simulink model "EZQ4sLStEnCtrl"  (R2018b)
settings: Solver=FixedStepDiscrete  StartTime=0.0  StopTime=20  FixedStep=0.01  RelTol=1e-3
undefined symbols (not defined in the file or in its folder): data, KeSMSw4SAcsMdSecRwLtStBkReclnRstTm_Val, KeSMSw4SSecRwLtStLgrstOtwdInwdClosePos1_Val, KeSMSw4SSecRwLtStLgrstUpwdDnwdClosePos1_Val, KeSMSw4SSecRwLtStLgrstUpwdDnwdClosePos2_Val, SecRwLtStBkReclnEn_Clear, SecRwLtStBkReclnEn_Set, SecRwLtStFtrstEn_Clear, SecRwLtStFtrstEn_Set, SecRwLtStFwdBkwdEn_Clear, SecRwLtStFwdBkwdEn_Set, SecRwLtStLgrstInwdOtwdEn_Clear, SecRwLtStLgrstInwdOtwdEn_Set, SecRwLtStLgrstUpwdDnwdEn_Clear, SecRwLtStLgrstUpwdDnwdEn_Set
libraries: simulink x1
settings Model: Creator=sn2xws  LastModifiedBy=sn2xws
settings Model: ModifiedHistory=|
  | 2023.8.1 V2.0.0 CR421790 增加模式21-26
  | 2023.10.17
  | V2.3.0 Bug 554442 4座2L便利下车，乘员离开座椅后，靠背位置没有从17%运动到50%
  | 在empty后面增加一个延时
settings DataIOCC: SaveFormat=StructureWithTime
settings OptimizationCC: DefaultParameterBehavior=Inlined  EnhancedBackFolding=on  PassReuseOutputArgsAs=Individual arguments  ZeroExternalMemoryAtStartup=off  ZeroInternalMemoryAtStartup=off  OptimizeBlockOrder=speed  DifferentSizesBufferReuse=on  OptimizationCustomize=off
settings DebuggingCC: ParameterTunabilityLossMsg=error
settings SFSimCC: MATLABDynamicMemAlloc=off
settings RTWCC: SystemTargetFile=autosar.tlc  GenCodeOnly=on  TemplateMakefile=ert_default_tmf  Description=AUTOSAR  GenerateReport=on  IncludeHyperlinkInReport=on  LaunchReport=on  GenerateTraceInfo=on  GenerateTraceReport=on  GenerateTraceReportSl=on  GenerateTraceReportSf=on  GenerateTraceReportEml=on  GenerateCodeMetricsReport=on
settings CodeAppCC: ForceParamTrailComments=on  IgnoreCustomStorageClasses=off  OperatorAnnotations=on  SimulinkDataObjDesc=on  SFDataObjDesc=on  InsertBlockDesc=on
settings STFCustomTargetCC: TargetLangStandard=C99 (ISO)  MultiwordLength=256  ParMdlRefBuildCompliant=on  CompOptLevelCompliant=on  IncludeMdlTerminateFcn=off  CombineOutputUpdateFcns=on  SuppressErrorStatus=on  ERTCustomFileBanners=on  SupportNonFinite=off  SupportComplex=off  SupportContinuousTime=off  SupportNonInlinedSFcns=off  RemoveResetFunc=on  MATLABClassNameForMDSCustomization=Simulink.SoftwareTarget.ERTCustomization  AutosarCompliant=on  UseToolchainInfoCompliant=on  LookupTableObjectStructAxisOrder=2,1,3,4,...  LUTObjectStructOrderEvenSpacing=Size,Table,Breakpoints  SystemTargetFile=autosar.tlc
settings ERTTargetCC: TargetLangStandard=C99 (ISO)  ConcurrentExecutionCompliant=off  IncludeMdlTerminateFcn=off  SuppressErrorStatus=on  SupportNonFinite=off  SupportComplex=off  ModelStepFunctionPrototypeControlCompliant=off  CPPClassGenCompliant=off  AutosarCompliant=on  LookupTableObjectStructAxisOrder=2,1,3,4,...  LUTObjectStructOrderEvenSpacing=Size,Table,Breakpoints  InlinedParameterPlacement=NonHierarchical  ERTCustomFileTemplate=example_file_process.tlc  ERTFilePackagingFormat=Compact

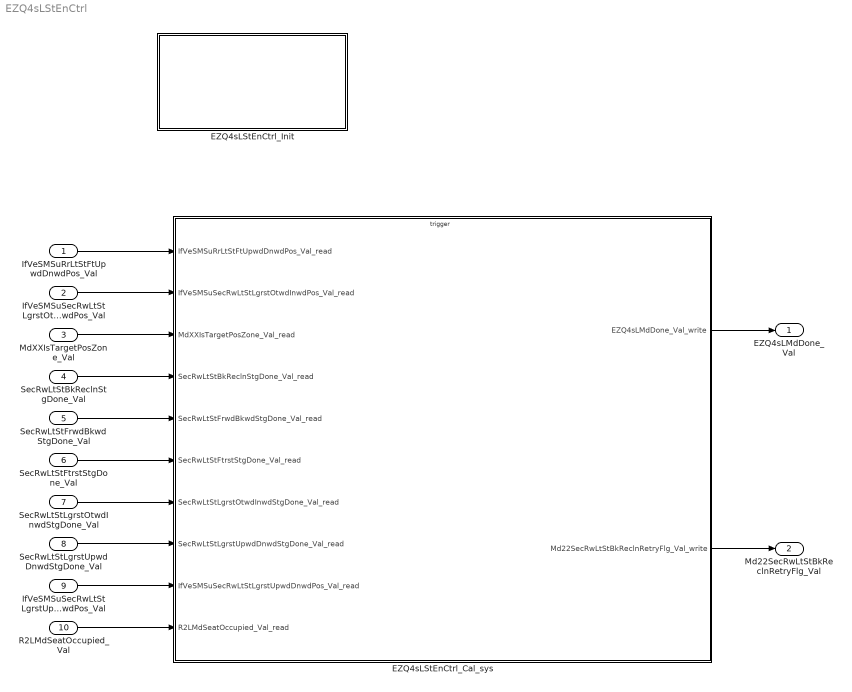
== system EZQ4sLStEnCtrl ==
  IfVeSMSuRrLtStFtUpwdDnwdPos_Val : Inport  OutDataTypeStr=uint16  PortDimensions=1
  IfVeSMSuSecRwLtStLgrstOtwdInwdPos_Val : Inport  Port=2  OutDataTypeStr=uint16  PortDimensions=1
  MdXXIsTargetPosZone_Val : Inport  Port=3  OutDataTypeStr=uint32  PortDimensions=1
  SecRwLtStBkReclnStgDone_Val : Inport  Port=4  OutDataTypeStr=boolean  PortDimensions=1
  SecRwLtStFrwdBkwdStgDone_Val : Inport  Port=5  OutDataTypeStr=boolean  PortDimensions=1
  SecRwLtStFtrstStgDone_Val : Inport  Port=6  OutDataTypeStr=boolean  PortDimensions=1
  SecRwLtStLgrstOtwdInwdStgDone_Val : Inport  Port=7  OutDataTypeStr=boolean  PortDimensions=1
  SecRwLtStLgrstUpwdDnwdStgDone_Val : Inport  Port=8  OutDataTypeStr=boolean  PortDimensions=1
  IfVeSMSuSecRwLtStLgrstUpwdDnwdPos_Val : Inport  Port=9  OutDataTypeStr=uint16  PortDimensions=1
  R2LMdSeatOccupied_Val : Inport  Port=10  OutDataTypeStr=boolean  PortDimensions=1
  EZQ4sLStEnCtrl_Cal_sys : Subsystem
  EZQ4sLStEnCtrl_Init : Subsystem
  EZQ4sLMdDone_Val : Outport  OutDataTypeStr=uint8  PortDimensions=1
  Md22SecRwLtStBkReclnRetryFlg_Val : Outport  Port=2  OutDataTypeStr=boolean  PortDimensions=1
  wires:
  IfVeSMSuRrLtStFtUpwdDnwdPos_Val/1 -> EZQ4sLStEnCtrl_Cal_sys/1(IfVeSMSuRrLtStFtUpwdDnwdPos_Val_read)
  IfVeSMSuSecRwLtStLgrstOtwdInwdPos_Val/1 -> EZQ4sLStEnCtrl_Cal_sys/2(IfVeSMSuSecRwLtStLgrstOtwdInwdPos_Val_read)
  MdXXIsTargetPosZone_Val/1 -> EZQ4sLStEnCtrl_Cal_sys/3(MdXXIsTargetPosZone_Val_read)
  SecRwLtStBkReclnStgDone_Val/1 -> EZQ4sLStEnCtrl_Cal_sys/4(SecRwLtStBkReclnStgDone_Val_read)
  SecRwLtStFrwdBkwdStgDone_Val/1 -> EZQ4sLStEnCtrl_Cal_sys/5(SecRwLtStFrwdBkwdStgDone_Val_read)
  SecRwLtStFtrstStgDone_Val/1 -> EZQ4sLStEnCtrl_Cal_sys/6(SecRwLtStFtrstStgDone_Val_read)
  SecRwLtStLgrstOtwdInwdStgDone_Val/1 -> EZQ4sLStEnCtrl_Cal_sys/7(SecRwLtStLgrstOtwdInwdStgDone_Val_read)
  SecRwLtStLgrstUpwdDnwdStgDone_Val/1 -> EZQ4sLStEnCtrl_Cal_sys/8(SecRwLtStLgrstUpwdDnwdStgDone_Val_read)
  EZQ4sLStEnCtrl_Cal_sys/1(EZQ4sLMdDone_Val_write) -> EZQ4sLMdDone_Val/1
  EZQ4sLStEnCtrl_Cal_sys/2(Md22SecRwLtStBkReclnRetryFlg_Val_write) -> Md22SecRwLtStBkReclnRetryFlg_Val/1
  IfVeSMSuSecRwLtStLgrstUpwdDnwdPos_Val/1 -> EZQ4sLStEnCtrl_Cal_sys/9(IfVeSMSuSecRwLtStLgrstUpwdDnwdPos_Val_read)
  R2LMdSeatOccupied_Val/1 -> EZQ4sLStEnCtrl_Cal_sys/10(R2LMdSeatOccupied_Val_read)

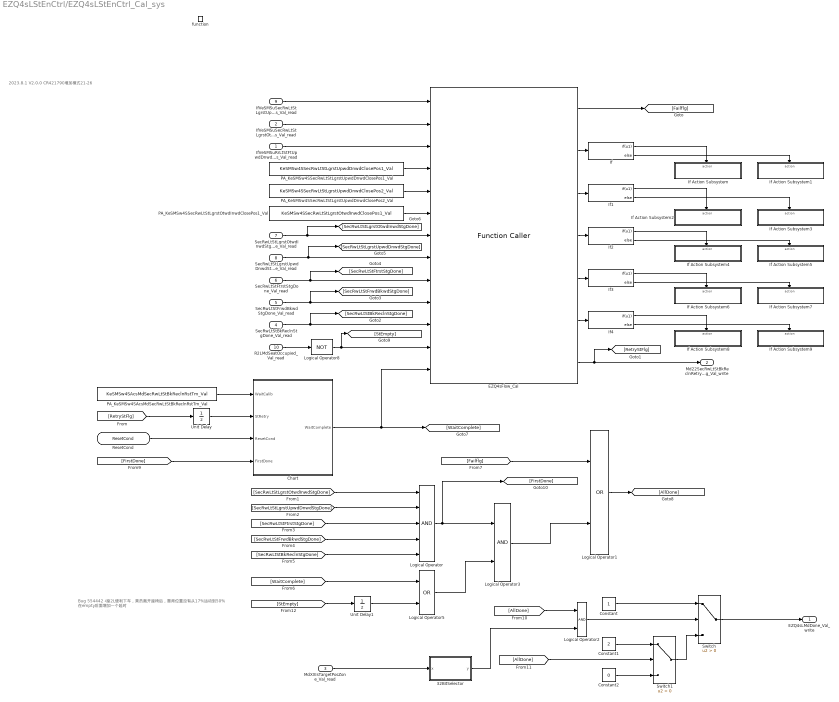
== system EZQ4sLStEnCtrl/EZQ4sLStEnCtrl_Cal_sys ==
  note: Bug 554442 4座2L便利下车，乘员离开座椅后，靠背位置没有从17%运动到50%
      | 在empty后面增加一个延时
  note: 2023.8.1 V2.0.0 CR421790 增加模式21-26
  IfVeSMSuRrLtStFtUpwdDnwdPos_Val_read : Inport
  IfVeSMSuSecRwLtStLgrstOtwdInwdPos_Val_read : Inport  Port=2
  MdXXIsTargetPosZone_Val_read : Inport  Port=3
  SecRwLtStBkReclnStgDone_Val_read : Inport  Port=4
  SecRwLtStFrwdBkwdStgDone_Val_read : Inport  Port=5
  SecRwLtStFtrstStgDone_Val_read : Inport  Port=6
  SecRwLtStLgrstOtwdInwdStgDone_Val_read : Inport  Port=7
  SecRwLtStLgrstUpwdDnwdStgDone_Val_read : Inport  Port=8
  IfVeSMSuSecRwLtStLgrstUpwdDnwdPos_Val_read : Inport  Port=9
  R2LMdSeatOccupied_Val_read : Inport  Port=10
  function : TriggerPort  TriggerType=function-call  IsSimulinkFunction=on  FunctionName=EZQ4sLStEnCtrl_Cal  VariantControl=(inherit)
  32BitSelector : Subsystem  mask(32 Bit Selector){BitNum=21}
      mask prompts: BitNum "Select Bit Number"
      mask help: Allows selection of a particular bit (0-31) out of a packed word up to 32 bits long. Output will be true if the bit number selected via the mask parameter is equal to one.
      mask TypeOptions BitNum: 0 | 1 | 2 | 3 | 4 | 5 | 6 | 7 | 8 | 9 | 10 | 11 | 12 | 13 | 14 | 15 | 16 | 17 | 18 | 19 | 20 | 21 | 22 | 23 | 24 | 25 | 26 | 27 | 28 | 29 | 30 | 31
      mask Display:
      | text(0.5, 0.8,'BIT','horizontalAlignment','center')
      | text(0.5, 0.5,'SELECTOR','horizontalAlignment','center')
      | text(0.5, 0.2,['-- Bit ',char(get_param(gcb,'BitNum')),' --'],'horizontalAlignment','center')
  Chart : Stateflow chart  TreatAsAtomicUnit=on
  Constant : Constant  OutDataTypeStr=uint8
  Constant1 : Constant  Value=2  OutDataTypeStr=uint8
  Constant2 : Constant  Value=0  OutDataTypeStr=uint8
  EZQ4sFlow_Cal : FunctionCaller  FunctionPrototype=[Failflg,LgrstInwdOtwdEn,LgrstUpwdDnwdEn,FtrstEn,FrwdBkwdEn,BkReclnEn,RetryStFlg] = EZQ4sFlow_Cal(LgrstUpwdDnwdPos,LgrstOtwdInwdPos,FtUpwdDnwdPos,CloseDnwdPos1,CloseDnwdPos2,CloseOtwdPos1,LgrstInwdStgDone,LgrstUpwdStgDone,FtrstStgDone,FrwdBkwdStgDone,BkReclnStgDone,StEmpty,WaitComplete)  InputArgumentSpecifications=uint16(1), uint16(1), uint16(1), uint16(1), uint16(1), uint16(1), boolean(true), boolean(true), boolean(true), boolean(true), boolean(true), boolean(true), boolean(true)  OutputArgumentSpecifications=boolean(true), boolean(true), boolean(true), boolean(true), boolean(true), boolean(true), boolean(true)
  If{,1..4} (5 alike) : If  IfExpression=u1
  If Action Subsystem : Subsystem  TreatAsAtomicUnit=on
  If Action Subsystem1 : Subsystem  TreatAsAtomicUnit=on
  If Action Subsystem2 : Subsystem  TreatAsAtomicUnit=on
  If Action Subsystem3 : Subsystem  TreatAsAtomicUnit=on
  If Action Subsystem4 : Subsystem  TreatAsAtomicUnit=on
  If Action Subsystem5 : Subsystem  TreatAsAtomicUnit=on
  If Action Subsystem6 : Subsystem  TreatAsAtomicUnit=on
  If Action Subsystem7 : Subsystem  TreatAsAtomicUnit=on
  If Action Subsystem8 : Subsystem  TreatAsAtomicUnit=on
  If Action Subsystem9 : Subsystem  TreatAsAtomicUnit=on
  Logical Operator : Logic  Inputs=5  AllPortsSameDT=off  OutDataTypeStr=boolean
  Logical Operator1 : Logic  Operator=OR  AllPortsSameDT=off  OutDataTypeStr=boolean
  Logical Operator2 : Logic  AllPortsSameDT=off  OutDataTypeStr=boolean
  Logical Operator3 : Logic  AllPortsSameDT=off  OutDataTypeStr=boolean
  Logical Operator5 : Logic  Operator=OR  AllPortsSameDT=off  OutDataTypeStr=boolean
  Logical Operator8 : Logic  Operator=NOT  AllPortsSameDT=off  OutDataTypeStr=boolean
  PA_KeSMSw4SAcsMdSecRwLtStBkReclnRstTm_Val : Constant  Value=KeSMSw4SAcsMdSecRwLtStBkReclnRstTm_Val
  PA_KeSMSw4SSecRwLtStLgrstOtwdInwdClosePos1_Val : Constant  Value=KeSMSw4SSecRwLtStLgrstOtwdInwdClosePos1_Val
  PA_KeSMSw4SSecRwLtStLgrstUpwdDnwdClosePos1_Val : Constant  Value=KeSMSw4SSecRwLtStLgrstUpwdDnwdClosePos1_Val
  PA_KeSMSw4SSecRwLtStLgrstUpwdDnwdClosePos2_Val : Constant  Value=KeSMSw4SSecRwLtStLgrstUpwdDnwdClosePos2_Val
  Switch : Switch  Criteria=u2 > Threshold
  Switch1 : Switch  Criteria=u2 > Threshold
  Unit Delay : UnitDelay  SampleTime=-1
  Unit Delay1 : UnitDelay  SampleTime=-1
  ResetCond : ArgIn  OutDataTypeStr=boolean  ArgumentName=ResetCond
  EZQ4sLMdDone_Val_write : Outport
      settings: EnsureOutportIsVirtual=on
  Md22SecRwLtStBkReclnRetryFlg_Val_write : Outport  Port=2
      settings: EnsureOutportIsVirtual=on
  wires:
  EZQ4sFlow_Cal/7 -> [RetryStFlg], Md22SecRwLtStBkReclnRetryFlg_Val_write/1
  IfVeSMSuRrLtStFtUpwdDnwdPos_Val_read/1 -> EZQ4sFlow_Cal/3
  IfVeSMSuSecRwLtStLgrstOtwdInwdPos_Val_read/1 -> EZQ4sFlow_Cal/2
  SecRwLtStLgrstOtwdInwdStgDone_Val_read/1 -> [SecRwLtStLgrstOtwdInwdStgDone], EZQ4sFlow_Cal/7
  SecRwLtStLgrstUpwdDnwdStgDone_Val_read/1 -> [SecRwLtStLgrstUpwdDnwdStgDone], EZQ4sFlow_Cal/8
  SecRwLtStFtrstStgDone_Val_read/1 -> [SecRwLtStFtrstStgDone], EZQ4sFlow_Cal/9
  SecRwLtStFrwdBkwdStgDone_Val_read/1 -> [SecRwLtStFrwdBkwdStgDone], EZQ4sFlow_Cal/10
  SecRwLtStBkReclnStgDone_Val_read/1 -> [SecRwLtStBkReclnStgDone], EZQ4sFlow_Cal/11
  IfVeSMSuSecRwLtStLgrstUpwdDnwdPos_Val_read/1 -> EZQ4sFlow_Cal/1
  PA_KeSMSw4SSecRwLtStLgrstUpwdDnwdClosePos1_Val/1 -> EZQ4sFlow_Cal/4
  PA_KeSMSw4SSecRwLtStLgrstUpwdDnwdClosePos2_Val/1 -> EZQ4sFlow_Cal/5
  PA_KeSMSw4SSecRwLtStLgrstOtwdInwdClosePos1_Val/1 -> EZQ4sFlow_Cal/6
  EZQ4sFlow_Cal/1 -> [Failflg]
  R2LMdSeatOccupied_Val_read/1 -> Logical Operator8/1
  Chart/1(WaitComplete) -> [WaitComplete], EZQ4sFlow_Cal/13
  EZQ4sFlow_Cal/2 -> If/1
  EZQ4sFlow_Cal/3 -> If1/1
  EZQ4sFlow_Cal/4 -> If2/1
  EZQ4sFlow_Cal/5 -> If3/1
  EZQ4sFlow_Cal/6 -> If4/1
  PA_KeSMSw4SAcsMdSecRwLtStBkReclnRstTm_Val/1 -> Chart/1(WaitCalib)
  Unit Delay/1 -> Chart/2(StRetry)
  [RetryStFlg] -> Unit Delay/1
  [SecRwLtStLgrstOtwdInwdStgDone] -> Logical Operator/1
  [SecRwLtStLgrstUpwdDnwdStgDone] -> Logical Operator/2
  [SecRwLtStFtrstStgDone] -> Logical Operator/3
  [SecRwLtStFrwdBkwdStgDone] -> Logical Operator/4
  [SecRwLtStBkReclnStgDone] -> Logical Operator/5
  [Failflg] -> Logical Operator1/1
  Logical Operator1/1 -> [AllDone]
  Constant1/1 -> Switch1/1
  Constant/1 -> Switch/1
  32BitSelector/1(y) -> Logical Operator2/2
  Switch1/1 -> Switch/3
  MdXXIsTargetPosZone_Val_read/1 -> 32BitSelector/1(x)
  Logical Operator2/1 -> Switch/2
  Constant2/1 -> Switch1/3
  Switch/1 -> EZQ4sLMdDone_Val_write/1
  [AllDone] -> Logical Operator2/1
  [AllDone] -> Switch1/2
  ResetCond/1 -> Chart/3(ResetCond)
  If/1 -> If Action Subsystem/Action
  If/2 -> If Action Subsystem1/Action
  If1/1 -> If Action Subsystem2/Action
  If1/2 -> If Action Subsystem3/Action
  If2/1 -> If Action Subsystem4/Action
  If2/2 -> If Action Subsystem5/Action
  If3/2 -> If Action Subsystem7/Action
  If3/1 -> If Action Subsystem6/Action
  If4/1 -> If Action Subsystem8/Action
  If4/2 -> If Action Subsystem9/Action
  Logical Operator3/1 -> Logical Operator1/2
  Logical Operator5/1 -> Logical Operator3/2
  [WaitComplete] -> Logical Operator5/1
  [StEmpty] -> Unit Delay1/1
  [FirstDone] -> Chart/4(FirstDone)
  Logical Operator/1 -> Logical Operator3/1, [FirstDone]
  Logical Operator8/1 -> EZQ4sFlow_Cal/12, [StEmpty]
  Unit Delay1/1 -> Logical Operator5/2

== system EZQ4sLStEnCtrl/EZQ4sLStEnCtrl_Init ==
  Event Listener : EventListener  EventName=reset

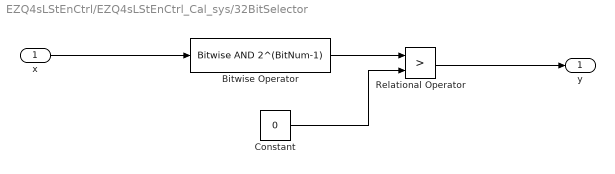
== system EZQ4sLStEnCtrl/EZQ4sLStEnCtrl_Cal_sys/32BitSelector ==
  x : Inport
  Bitwise Operator : simulink/Logic and Bit Operations/Bitwise Operator  logicop=AND  UseBitMask=on  BitMask=2^(BitNum-1)  BitMaskRealWorld=Stored Integer
  Constant : Constant  Value=0  OutDataTypeStr=uint32
  Relational Operator : RelationalOperator  Operator=>  OutDataTypeStr=boolean  RndMeth=Simplest
  y : Outport
  wires:
  Relational Operator/1 -> y/1
  Constant/1 -> Relational Operator/2
  x/1 -> Bitwise Operator/1
  Bitwise Operator/1 -> Relational Operator/1

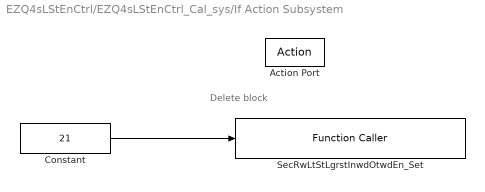
== system EZQ4sLStEnCtrl/EZQ4sLStEnCtrl_Cal_sys/If Action Subsystem ==
  note: Delete block
  Action Port : ActionPort  ActionType=then
  Constant : Constant  Value=21  OutDataTypeStr=uint8
  SecRwLtStLgrstInwdOtwdEn_Set : FunctionCaller  FunctionPrototype=SecRwLtStLgrstInwdOtwdEn_Set(data)  InputArgumentSpecifications=uint8(1)
  wires:
  Constant/1 -> SecRwLtStLgrstInwdOtwdEn_Set/1

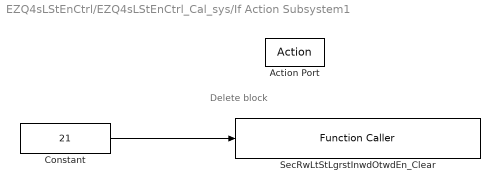
== system EZQ4sLStEnCtrl/EZQ4sLStEnCtrl_Cal_sys/If Action Subsystem1 ==
  note: Delete block
  Action Port : ActionPort  ActionType=else
  Constant : Constant  Value=21  OutDataTypeStr=uint8
  SecRwLtStLgrstInwdOtwdEn_Clear : FunctionCaller  FunctionPrototype=SecRwLtStLgrstInwdOtwdEn_Clear(data)  InputArgumentSpecifications=uint8(1)
  wires:
  Constant/1 -> SecRwLtStLgrstInwdOtwdEn_Clear/1

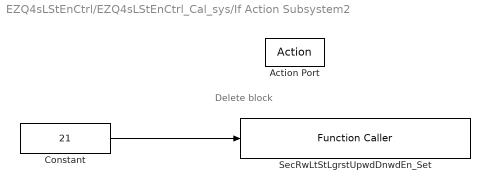
== system EZQ4sLStEnCtrl/EZQ4sLStEnCtrl_Cal_sys/If Action Subsystem2 ==
  note: Delete block
  Action Port : ActionPort  ActionType=then
  Constant : Constant  Value=21  OutDataTypeStr=uint8
  SecRwLtStLgrstUpwdDnwdEn_Set : FunctionCaller  FunctionPrototype=SecRwLtStLgrstUpwdDnwdEn_Set(data)  InputArgumentSpecifications=uint8(1)
  wires:
  Constant/1 -> SecRwLtStLgrstUpwdDnwdEn_Set/1

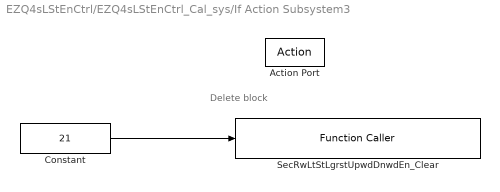
== system EZQ4sLStEnCtrl/EZQ4sLStEnCtrl_Cal_sys/If Action Subsystem3 ==
  note: Delete block
  Action Port : ActionPort  ActionType=else
  Constant : Constant  Value=21  OutDataTypeStr=uint8
  SecRwLtStLgrstUpwdDnwdEn_Clear : FunctionCaller  FunctionPrototype=SecRwLtStLgrstUpwdDnwdEn_Clear(data)  InputArgumentSpecifications=uint8(1)
  wires:
  Constant/1 -> SecRwLtStLgrstUpwdDnwdEn_Clear/1

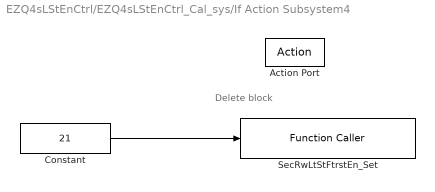
== system EZQ4sLStEnCtrl/EZQ4sLStEnCtrl_Cal_sys/If Action Subsystem4 ==
  note: Delete block
  Action Port : ActionPort  ActionType=then
  Constant : Constant  Value=21  OutDataTypeStr=uint8
  SecRwLtStFtrstEn_Set : FunctionCaller  FunctionPrototype=SecRwLtStFtrstEn_Set(data)  InputArgumentSpecifications=uint8(1)
  wires:
  Constant/1 -> SecRwLtStFtrstEn_Set/1

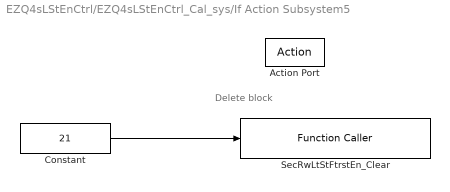
== system EZQ4sLStEnCtrl/EZQ4sLStEnCtrl_Cal_sys/If Action Subsystem5 ==
  note: Delete block
  Action Port : ActionPort  ActionType=else
  Constant : Constant  Value=21  OutDataTypeStr=uint8
  SecRwLtStFtrstEn_Clear : FunctionCaller  FunctionPrototype=SecRwLtStFtrstEn_Clear(data)  InputArgumentSpecifications=uint8(1)
  wires:
  Constant/1 -> SecRwLtStFtrstEn_Clear/1

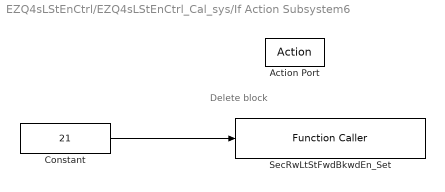
== system EZQ4sLStEnCtrl/EZQ4sLStEnCtrl_Cal_sys/If Action Subsystem6 ==
  note: Delete block
  Action Port : ActionPort  ActionType=then
  Constant : Constant  Value=21  OutDataTypeStr=uint8
  SecRwLtStFwdBkwdEn_Set : FunctionCaller  FunctionPrototype=SecRwLtStFwdBkwdEn_Set(data)  InputArgumentSpecifications=uint8(1)
  wires:
  Constant/1 -> SecRwLtStFwdBkwdEn_Set/1

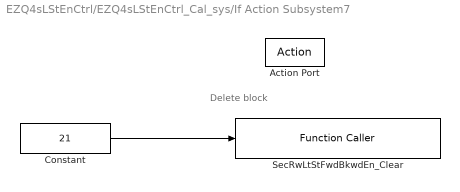
== system EZQ4sLStEnCtrl/EZQ4sLStEnCtrl_Cal_sys/If Action Subsystem7 ==
  note: Delete block
  Action Port : ActionPort  ActionType=else
  Constant : Constant  Value=21  OutDataTypeStr=uint8
  SecRwLtStFwdBkwdEn_Clear : FunctionCaller  FunctionPrototype=SecRwLtStFwdBkwdEn_Clear(data)  InputArgumentSpecifications=uint8(1)
  wires:
  Constant/1 -> SecRwLtStFwdBkwdEn_Clear/1

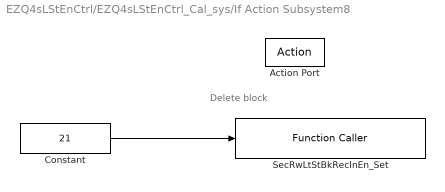
== system EZQ4sLStEnCtrl/EZQ4sLStEnCtrl_Cal_sys/If Action Subsystem8 ==
  note: Delete block
  Action Port : ActionPort  ActionType=then
  Constant : Constant  Value=21  OutDataTypeStr=uint8
  SecRwLtStBkReclnEn_Set : FunctionCaller  FunctionPrototype=SecRwLtStBkReclnEn_Set(data)  InputArgumentSpecifications=uint8(1)
  wires:
  Constant/1 -> SecRwLtStBkReclnEn_Set/1

== system EZQ4sLStEnCtrl/EZQ4sLStEnCtrl_Cal_sys/If Action Subsystem9 ==
  note: Delete block
  Action Port : ActionPort  ActionType=else
  Constant : Constant  Value=21  OutDataTypeStr=uint8
  SecRwLtStBkReclnEn_Clear : FunctionCaller  FunctionPrototype=SecRwLtStBkReclnEn_Clear(data)  InputArgumentSpecifications=uint8(1)
  wires:
  Constant/1 -> SecRwLtStBkReclnEn_Clear/1

== stateflow chart EZQ4sLStEnCtrl/EZQ4sLStEnCtrl_Cal_sys/Chart ==
  (default) -> (junction 16)
  (junction 16) -> (junction 18) [order 1] : [ResetCond]
  (junction 16) -> (junction 21) [order 2]
  (junction 18) -> (junction 23) : {
      | WaitCnt = 0;
      | WaitComplete=false;
      | }
  (junction 23) -> (junction 21)
  (junction 21) -> (junction 26)
  (junction 26) -> (junction 28) [order 1] : [FirstDone]
  (junction 26) -> (junction 30) [order 2]
  (junction 28) -> (junction 32) : {WaitCnt = WaitCnt +1;}
  (junction 32) -> (junction 30)
  (junction 30) -> (junction 5)
  (junction 5) -> (junction 7) [order 1] : [StRetry||WaitCnt>WaitCalib]
  (junction 5) -> (junction 11) [order 2]
  (junction 7) -> (junction 9) : {WaitComplete=true;}
  (junction 9) -> (junction 11)
  (junction 11) -> (junction 14)
  data: WaitCnt local uint16; WaitCalib input; WaitComplete output boolean; StRetry input; ResetCond input; FirstDone input
